simulink model "Simulink_Simulation"  (Simulink 10.1)
settings: Solver=ode23t  StartTime=0.0  StopTime=0.08  RelTol=1e-3  EnableMultiTasking=on
libraries: powerlib x10, powerlib_meascontrol x1
settings Model: Creator=asus1  LastModifiedBy=x64
settings DataIOCC: LimitDataPoints=on
settings DebuggingCC: UnderspecifiedInitializationDetection=Simplified  MergeDetectMultiDrivingBlocksExec=error  SolverPrmCheckMsg=warning
settings GRTTargetCC: CombineOutputUpdateFcns=on  GRTInterface=off
settings ConfigComp: CovSFcnEnable=off
settings SimscapeCC: SimscapeNormalizeSystem=off

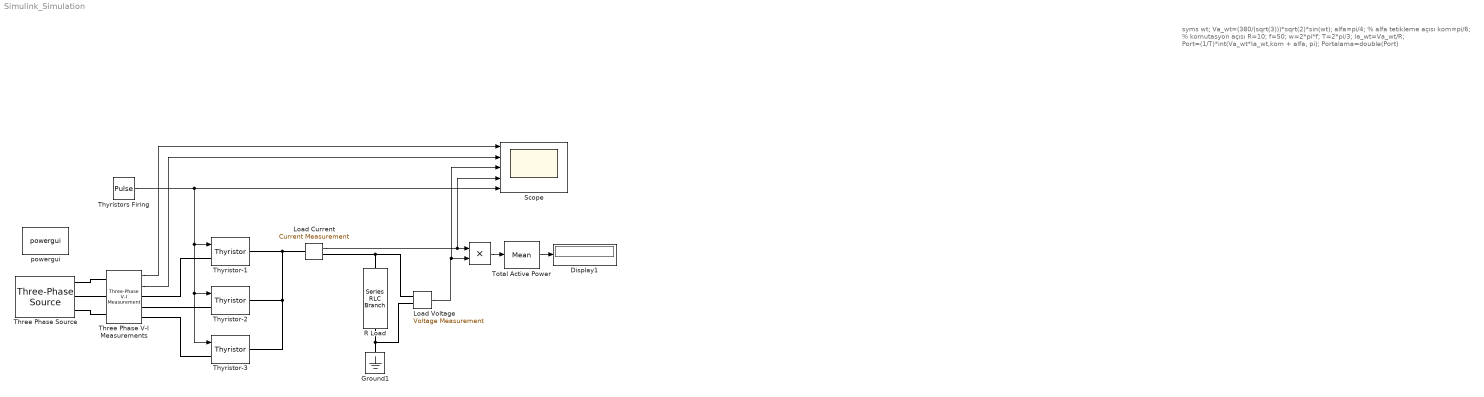
== system Simulink_Simulation ==
  note: syms wt;
      | Va_wt=(380/(sqrt(3)))*sqrt(2)*sin(wt);
      | alfa=pi/4; % alfa tetikleme açısı
      | kom=pi/6; % komutasyon açısı
      | R=10;
      | f=50;
      | w=2*pi*f;
      | T=2*pi/3;
      | Ia_wt=Va_wt/R;
      | Port=(1/T)*int(Va_wt*Ia_wt,kom + alfa, pi);
      | Portalama=double(Port)
  "    " : Product
  Display1 : Display
      settings: Format=bank
  Ground1 : powerlib/Elements/Ground  LConnTagsString=a
  Load Current : powerlib/Measurements/Current Measurement  PhasorSimulation=off  OutputType=Complex  PSBequivalent=0
  Load Voltage : powerlib/Measurements/Voltage Measurement  PhasorSimulation=off  OutputType=Complex  PSBequivalent=0
  "R Load " : powerlib/Elements/Series RLC Branch  LConnTagsString=__new0  RConnTagsString=__new0  BranchType=R  Resistance=10  Inductance=1e-3  SetiL0=off  InitialCurrent=0  Capacitance=1e-6  Setx0=off  InitialVoltage=0  Measurements=None
  Scope : Scope  NumInputPorts=5
  Three Phase V-I Measurements : powerlib/Measurements/Three-Phase V-I Measurement  VoltageMeasurement=phase-to-ground  SetLabelV=off  LabelV=Vabc  Vpu=off  VpuLL=off  CurrentMeasurement=yes  SetLabelI=off  LabelI=Iabc  Ipu=off  Pbase=100e6  Vbase=500e3  OutputType=Complex  PhasorSimulation=off  PSBequivalent=0
  Three Phase Source : powerlib/Electrical Sources/Three-Phase Source  InternalConnection=Yg  VoltagePhases=off  Voltage=380  PhaseAngle=0  Voltage_phases=[25e3 25e3 25e3]/sqrt(3)  PhaseAngles_phases=[0 -120 +120]  Frequency=50  NonIdealSource=on  SpecifyImpedance=on  Resistance=0.8929  Inductance=16.58e-3  ShortCircuitLevel=100e6  BaseVoltage=380  XRratio=7  BusType=swing  Pref=0  Qref=0  Prefabc=[10e3, 10e3, 10e3]  Qrefabc=[0, 0, 0]  Qmin=-inf  Qmax=inf
  Thyristor-1 : powerlib/Power Electronics/Thyristor  Ron=0.00001  Lon=0  Vf=0  IC=0  Rs=5000  Cs=250e-6  Measurements=off
  Thyristor-2 : powerlib/Power Electronics/Thyristor  Ron=0.00001  Lon=0  Vf=0  IC=0  Rs=5000  Cs=250e-6  Measurements=off
  Thyristor-3 : powerlib/Power Electronics/Thyristor  Ron=0.00001  Lon=0  Vf=0  IC=0  Rs=5000  Cs=250e-6  Measurements=off
  Thyristors Firing : DiscretePulseGenerator  PulseType=Time based  Amplitude=5  Period=0.02/3  PulseWidth=5  PhaseDelay=0.0041667
  Total Active Power : powerlib_meascontrol/Measurements/Mean  Freq=50  Vinit=0  Ts=0
  powergui : powerlib/powergui  Priority=1  SimulationMode=Discrete  SampleTime=5e-6  frequency=60  Iterations=50  frequencyindice=50  Pbase=100e6  ErrMax=1e-4  UnitsV=kV  UnitsW=MW  buscounter=0  FunctionMessages=off  echomessages=off  EnableUseOfTLC=off  CurrentSourceSwitches=off  DisableSnubberDevices=off  DisableRonSwitches=off  DisableVfSwitches=off  DisplayEquations=off  AutomaticDiscreteSolvers=off  SolverType=Tustin  Interpol=off  ExternalGateDelay=off  methode=off  Ts=100  x0status=blocks  SPID=off  SwTol=0  HookPort=off  NonlinearTolerance=1e-4  nMaxIteration=100  ContinueOnMaxIteration=off  RestoreLinks=warning  ResistiveCurrentMeasurement=off  Frange=[0:2:500]  Ylog=off  Xlog=on  ShowGrid=off  save=off  variable=ZData  structure=0  ZoomFFT=off  StartTime=0.0  cycles=1  DisplayStyle=1  fundamental=60  FreqAxis=off  MaxFrequency=1000  frequencyindicesteady=1  RmsSteady=1  display=off
  wires:
  "    "/1 -> Total Active Power/1
  Total Active Power/1 -> Display1/1
  Thyristors Firing/1 -> Thyristor-3/1, Thyristor-2/1, Thyristor-1/1, Scope/5
  Load Current/1 -> Scope/4, "    "/1
  Load Voltage/1 -> Scope/3, "    "/2
  Three Phase V-I Measurements/1 -> Scope/1
  Three Phase V-I Measurements/2 -> Scope/2
  connections:
  "R Load "/RConn1 -- Load Voltage/LConn2 -- Ground1/LConn1
  Three Phase Source/RConn3 -- Three Phase V-I Measurements/LConn3
  Three Phase Source/RConn2 -- Three Phase V-I Measurements/LConn2
  Three Phase Source/RConn1 -- Three Phase V-I Measurements/LConn1
  Three Phase V-I Measurements/RConn3 -- Thyristor-3/LConn1
  Three Phase V-I Measurements/RConn2 -- Thyristor-2/LConn1
  Three Phase V-I Measurements/RConn1 -- Thyristor-1/LConn1
  Load Current/RConn1 -- Load Voltage/LConn1 -- "R Load "/LConn1
  Thyristor-1/RConn1 -- Load Current/LConn1 -- Thyristor-2/RConn1 -- Thyristor-3/RConn1
